simulink model "dsp48macro_mult35x35"  (Simulink 7.6)
settings: Solver=ode45  StartTime=0.0  StopTime=100.0  RelTol=1e-3
undefined symbols (not defined in the file): xlipgetpartsetting
libraries: xbsIndex_r4 x39, xbsCopyrightNotice_r4 x1
(part 2 of 2)

== system dsp48macro_mult35x35/More Info ==

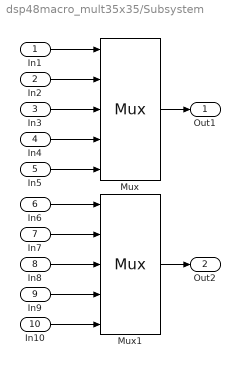
== system dsp48macro_mult35x35/Subsystem ==
  In1 : Inport
  In2 : Inport  Port=2
  In3 : Inport  Port=3
  In4 : Inport  Port=4
  In5 : Inport  Port=5
  In6 : Inport  Port=6
  In7 : Inport  Port=7
  In8 : Inport  Port=8
  In9 : Inport  Port=9
  In10 : Inport  Port=10
  Mux : xbsIndex_r4/Mux  inputs=4  en=off  latency=0  precision=Full  arith_type=Unsigned  n_bits=16  bin_pt=14  quantization=Truncate  overflow=Wrap  dbl_ovrd=off  block_type=mux
      settings: block_version=11.4
  Mux1 : xbsIndex_r4/Mux  inputs=4  en=off  latency=0  precision=Full  arith_type=Unsigned  n_bits=16  bin_pt=14  quantization=Truncate  overflow=Wrap  dbl_ovrd=off  block_type=mux
      settings: block_version=11.4
  Out1 : Outport
  Out2 : Outport  Port=2
  wires:
  In1/1 -> Mux/1
  In2/1 -> Mux/2
  In3/1 -> Mux/3
  Mux/1 -> Out1/1
  In4/1 -> Mux/4
  In5/1 -> Mux/5
  In6/1 -> Mux1/1
  In7/1 -> Mux1/2
  In8/1 -> Mux1/3
  Mux1/1 -> Out2/1
  In9/1 -> Mux1/4
  In10/1 -> Mux1/5
